simulink model "gm_fourxfour_designfxdpt_givens_vnl"  (R2018b)
settings: Solver=FixedStepDiscrete  StartTime=0.0  StopTime=0.18e-6  RelTol=1e-3
InitFcn:
  | if isempty(which('mylib'))
  |      tmp = fileparts(which(bdroot));
  |      run(fullfile(fileparts(tmp), '5-Utilities', 'addPathsPfcHw.m'));
  | end
  | 
  | data_types_givens
StopFcn:
  | GivensSim_Stop
undefined symbols (not defined in the file or in its folder): f
libraries: simulink x28, mylib x14
(part 2 of 4)

== system gm_fourxfour_designfxdpt_givens_vnl/Compare/Assert_R_11_i ==
  cosim : Inport
  dut : Inport  Port=2
  AssertEq : Assertion  StopWhenAssertionFail=off
  Compare To Zero : simulink/Logic and Bit Operations/Compare To Zero  relop===  OutDataTypeStr=boolean
  Relational Operator : RelationalOperator  Operator===  OutDataTypeStr=boolean  RndMeth=Nearest
  compare: R_11_i : Scope  NumInputPorts=3
  wires:
  Compare To Zero/1 -> compare: R_11_i/3  "err"
  Relational Operator/1 -> Compare To Zero/1, AssertEq/1
  cosim/1 -> compare: R_11_i/1, Relational Operator/1  "cosim"
  dut/1 -> compare: R_11_i/2, Relational Operator/2  "dut ref"

== system gm_fourxfour_designfxdpt_givens_vnl/Compare/Assert_R_11_r ==
  cosim : Inport
  dut : Inport  Port=2
  AssertEq : Assertion  StopWhenAssertionFail=off
  Compare To Zero : simulink/Logic and Bit Operations/Compare To Zero  relop===  OutDataTypeStr=boolean
  Relational Operator : RelationalOperator  Operator===  OutDataTypeStr=boolean  RndMeth=Nearest
  compare: R_11_r : Scope  NumInputPorts=3
  wires:
  Compare To Zero/1 -> compare: R_11_r/3  "err"
  Relational Operator/1 -> Compare To Zero/1, AssertEq/1
  cosim/1 -> compare: R_11_r/1, Relational Operator/1  "cosim"
  dut/1 -> compare: R_11_r/2, Relational Operator/2  "dut ref"

== system gm_fourxfour_designfxdpt_givens_vnl/Compare/Assert_R_12_i ==
  cosim : Inport
  dut : Inport  Port=2
  AssertEq : Assertion  StopWhenAssertionFail=off
  Compare To Zero : simulink/Logic and Bit Operations/Compare To Zero  relop===  OutDataTypeStr=boolean
  Relational Operator : RelationalOperator  Operator===  OutDataTypeStr=boolean  RndMeth=Nearest
  compare: R_12_i : Scope  NumInputPorts=3
  wires:
  Compare To Zero/1 -> compare: R_12_i/3  "err"
  Relational Operator/1 -> Compare To Zero/1, AssertEq/1
  cosim/1 -> compare: R_12_i/1, Relational Operator/1  "cosim"
  dut/1 -> compare: R_12_i/2, Relational Operator/2  "dut ref"

== system gm_fourxfour_designfxdpt_givens_vnl/Compare/Assert_R_12_r ==
  cosim : Inport
  dut : Inport  Port=2
  AssertEq : Assertion  StopWhenAssertionFail=off
  Compare To Zero : simulink/Logic and Bit Operations/Compare To Zero  relop===  OutDataTypeStr=boolean
  Relational Operator : RelationalOperator  Operator===  OutDataTypeStr=boolean  RndMeth=Nearest
  compare: R_12_r : Scope  NumInputPorts=3
  wires:
  Compare To Zero/1 -> compare: R_12_r/3  "err"
  Relational Operator/1 -> Compare To Zero/1, AssertEq/1
  cosim/1 -> compare: R_12_r/1, Relational Operator/1  "cosim"
  dut/1 -> compare: R_12_r/2, Relational Operator/2  "dut ref"

== system gm_fourxfour_designfxdpt_givens_vnl/Compare/Assert_R_13_i ==
  cosim : Inport
  dut : Inport  Port=2
  AssertEq : Assertion  StopWhenAssertionFail=off
  Compare To Zero : simulink/Logic and Bit Operations/Compare To Zero  relop===  OutDataTypeStr=boolean
  Relational Operator : RelationalOperator  Operator===  OutDataTypeStr=boolean  RndMeth=Nearest
  compare: R_13_i : Scope  NumInputPorts=3
  wires:
  Compare To Zero/1 -> compare: R_13_i/3  "err"
  Relational Operator/1 -> Compare To Zero/1, AssertEq/1
  cosim/1 -> compare: R_13_i/1, Relational Operator/1  "cosim"
  dut/1 -> compare: R_13_i/2, Relational Operator/2  "dut ref"

== system gm_fourxfour_designfxdpt_givens_vnl/Compare/Assert_R_13_r ==
  cosim : Inport
  dut : Inport  Port=2
  AssertEq : Assertion  StopWhenAssertionFail=off
  Compare To Zero : simulink/Logic and Bit Operations/Compare To Zero  relop===  OutDataTypeStr=boolean
  Relational Operator : RelationalOperator  Operator===  OutDataTypeStr=boolean  RndMeth=Nearest
  compare: R_13_r : Scope  NumInputPorts=3
  wires:
  Compare To Zero/1 -> compare: R_13_r/3  "err"
  Relational Operator/1 -> Compare To Zero/1, AssertEq/1
  cosim/1 -> compare: R_13_r/1, Relational Operator/1  "cosim"
  dut/1 -> compare: R_13_r/2, Relational Operator/2  "dut ref"

== system gm_fourxfour_designfxdpt_givens_vnl/Compare/Assert_R_14_i ==
  cosim : Inport
  dut : Inport  Port=2
  AssertEq : Assertion  StopWhenAssertionFail=off
  Compare To Zero : simulink/Logic and Bit Operations/Compare To Zero  relop===  OutDataTypeStr=boolean
  Relational Operator : RelationalOperator  Operator===  OutDataTypeStr=boolean  RndMeth=Nearest
  compare: R_14_i : Scope  NumInputPorts=3
  wires:
  Compare To Zero/1 -> compare: R_14_i/3  "err"
  Relational Operator/1 -> Compare To Zero/1, AssertEq/1
  cosim/1 -> compare: R_14_i/1, Relational Operator/1  "cosim"
  dut/1 -> compare: R_14_i/2, Relational Operator/2  "dut ref"

== system gm_fourxfour_designfxdpt_givens_vnl/Compare/Assert_R_14_r ==
  cosim : Inport
  dut : Inport  Port=2
  AssertEq : Assertion  StopWhenAssertionFail=off
  Compare To Zero : simulink/Logic and Bit Operations/Compare To Zero  relop===  OutDataTypeStr=boolean
  Relational Operator : RelationalOperator  Operator===  OutDataTypeStr=boolean  RndMeth=Nearest
  compare: R_14_r : Scope  NumInputPorts=3
  wires:
  Compare To Zero/1 -> compare: R_14_r/3  "err"
  Relational Operator/1 -> Compare To Zero/1, AssertEq/1
  cosim/1 -> compare: R_14_r/1, Relational Operator/1  "cosim"
  dut/1 -> compare: R_14_r/2, Relational Operator/2  "dut ref"

== system gm_fourxfour_designfxdpt_givens_vnl/Compare/Assert_R_22_i ==
  cosim : Inport
  dut : Inport  Port=2
  AssertEq : Assertion  StopWhenAssertionFail=off
  Compare To Zero : simulink/Logic and Bit Operations/Compare To Zero  relop===  OutDataTypeStr=boolean
  Relational Operator : RelationalOperator  Operator===  OutDataTypeStr=boolean  RndMeth=Nearest
  compare: R_22_i : Scope  NumInputPorts=3
  wires:
  Compare To Zero/1 -> compare: R_22_i/3  "err"
  Relational Operator/1 -> Compare To Zero/1, AssertEq/1
  cosim/1 -> compare: R_22_i/1, Relational Operator/1  "cosim"
  dut/1 -> compare: R_22_i/2, Relational Operator/2  "dut ref"

== system gm_fourxfour_designfxdpt_givens_vnl/Compare/Assert_R_22_r ==
  cosim : Inport
  dut : Inport  Port=2
  AssertEq : Assertion  StopWhenAssertionFail=off
  Compare To Zero : simulink/Logic and Bit Operations/Compare To Zero  relop===  OutDataTypeStr=boolean
  Relational Operator : RelationalOperator  Operator===  OutDataTypeStr=boolean  RndMeth=Nearest
  compare: R_22_r : Scope  NumInputPorts=3
  wires:
  Compare To Zero/1 -> compare: R_22_r/3  "err"
  Relational Operator/1 -> Compare To Zero/1, AssertEq/1
  cosim/1 -> compare: R_22_r/1, Relational Operator/1  "cosim"
  dut/1 -> compare: R_22_r/2, Relational Operator/2  "dut ref"

== system gm_fourxfour_designfxdpt_givens_vnl/Compare/Assert_R_23_i ==
  cosim : Inport
  dut : Inport  Port=2
  AssertEq : Assertion  StopWhenAssertionFail=off
  Compare To Zero : simulink/Logic and Bit Operations/Compare To Zero  relop===  OutDataTypeStr=boolean
  Relational Operator : RelationalOperator  Operator===  OutDataTypeStr=boolean  RndMeth=Nearest
  compare: R_23_i : Scope  NumInputPorts=3
  wires:
  Compare To Zero/1 -> compare: R_23_i/3  "err"
  Relational Operator/1 -> Compare To Zero/1, AssertEq/1
  cosim/1 -> compare: R_23_i/1, Relational Operator/1  "cosim"
  dut/1 -> compare: R_23_i/2, Relational Operator/2  "dut ref"

== system gm_fourxfour_designfxdpt_givens_vnl/Compare/Assert_R_23_r ==
  cosim : Inport
  dut : Inport  Port=2
  AssertEq : Assertion  StopWhenAssertionFail=off
  Compare To Zero : simulink/Logic and Bit Operations/Compare To Zero  relop===  OutDataTypeStr=boolean
  Relational Operator : RelationalOperator  Operator===  OutDataTypeStr=boolean  RndMeth=Nearest
  compare: R_23_r : Scope  NumInputPorts=3
  wires:
  Compare To Zero/1 -> compare: R_23_r/3  "err"
  Relational Operator/1 -> Compare To Zero/1, AssertEq/1
  cosim/1 -> compare: R_23_r/1, Relational Operator/1  "cosim"
  dut/1 -> compare: R_23_r/2, Relational Operator/2  "dut ref"

== system gm_fourxfour_designfxdpt_givens_vnl/Compare/Assert_R_24_i ==
  cosim : Inport
  dut : Inport  Port=2
  AssertEq : Assertion  StopWhenAssertionFail=off
  Compare To Zero : simulink/Logic and Bit Operations/Compare To Zero  relop===  OutDataTypeStr=boolean
  Relational Operator : RelationalOperator  Operator===  OutDataTypeStr=boolean  RndMeth=Nearest
  compare: R_24_i : Scope  NumInputPorts=3
  wires:
  Compare To Zero/1 -> compare: R_24_i/3  "err"
  Relational Operator/1 -> Compare To Zero/1, AssertEq/1
  cosim/1 -> compare: R_24_i/1, Relational Operator/1  "cosim"
  dut/1 -> compare: R_24_i/2, Relational Operator/2  "dut ref"

== system gm_fourxfour_designfxdpt_givens_vnl/Compare/Assert_R_24_r ==
  cosim : Inport
  dut : Inport  Port=2
  AssertEq : Assertion  StopWhenAssertionFail=off
  Compare To Zero : simulink/Logic and Bit Operations/Compare To Zero  relop===  OutDataTypeStr=boolean
  Relational Operator : RelationalOperator  Operator===  OutDataTypeStr=boolean  RndMeth=Nearest
  compare: R_24_r : Scope  NumInputPorts=3
  wires:
  Compare To Zero/1 -> compare: R_24_r/3  "err"
  Relational Operator/1 -> Compare To Zero/1, AssertEq/1
  cosim/1 -> compare: R_24_r/1, Relational Operator/1  "cosim"
  dut/1 -> compare: R_24_r/2, Relational Operator/2  "dut ref"

== system gm_fourxfour_designfxdpt_givens_vnl/Compare/Assert_R_33_i ==
  cosim : Inport
  dut : Inport  Port=2
  AssertEq : Assertion  StopWhenAssertionFail=off
  Compare To Zero : simulink/Logic and Bit Operations/Compare To Zero  relop===  OutDataTypeStr=boolean
  Relational Operator : RelationalOperator  Operator===  OutDataTypeStr=boolean  RndMeth=Nearest
  compare: R_33_i : Scope  NumInputPorts=3
  wires:
  Compare To Zero/1 -> compare: R_33_i/3  "err"
  Relational Operator/1 -> Compare To Zero/1, AssertEq/1
  cosim/1 -> compare: R_33_i/1, Relational Operator/1  "cosim"
  dut/1 -> compare: R_33_i/2, Relational Operator/2  "dut ref"

== system gm_fourxfour_designfxdpt_givens_vnl/Compare/Assert_R_33_r ==
  cosim : Inport
  dut : Inport  Port=2
  AssertEq : Assertion  StopWhenAssertionFail=off
  Compare To Zero : simulink/Logic and Bit Operations/Compare To Zero  relop===  OutDataTypeStr=boolean
  Relational Operator : RelationalOperator  Operator===  OutDataTypeStr=boolean  RndMeth=Nearest
  compare: R_33_r : Scope  NumInputPorts=3
  wires:
  Compare To Zero/1 -> compare: R_33_r/3  "err"
  Relational Operator/1 -> Compare To Zero/1, AssertEq/1
  cosim/1 -> compare: R_33_r/1, Relational Operator/1  "cosim"
  dut/1 -> compare: R_33_r/2, Relational Operator/2  "dut ref"

== system gm_fourxfour_designfxdpt_givens_vnl/Compare/Assert_R_34_i ==
  cosim : Inport
  dut : Inport  Port=2
  AssertEq : Assertion  StopWhenAssertionFail=off
  Compare To Zero : simulink/Logic and Bit Operations/Compare To Zero  relop===  OutDataTypeStr=boolean
  Relational Operator : RelationalOperator  Operator===  OutDataTypeStr=boolean  RndMeth=Nearest
  compare: R_34_i : Scope  NumInputPorts=3
  wires:
  Compare To Zero/1 -> compare: R_34_i/3  "err"
  Relational Operator/1 -> Compare To Zero/1, AssertEq/1
  cosim/1 -> compare: R_34_i/1, Relational Operator/1  "cosim"
  dut/1 -> compare: R_34_i/2, Relational Operator/2  "dut ref"

== system gm_fourxfour_designfxdpt_givens_vnl/Compare/Assert_R_34_r ==
  cosim : Inport
  dut : Inport  Port=2
  AssertEq : Assertion  StopWhenAssertionFail=off
  Compare To Zero : simulink/Logic and Bit Operations/Compare To Zero  relop===  OutDataTypeStr=boolean
  Relational Operator : RelationalOperator  Operator===  OutDataTypeStr=boolean  RndMeth=Nearest
  compare: R_34_r : Scope  NumInputPorts=3
  wires:
  Compare To Zero/1 -> compare: R_34_r/3  "err"
  Relational Operator/1 -> Compare To Zero/1, AssertEq/1
  cosim/1 -> compare: R_34_r/1, Relational Operator/1  "cosim"
  dut/1 -> compare: R_34_r/2, Relational Operator/2  "dut ref"

== system gm_fourxfour_designfxdpt_givens_vnl/Compare/Assert_R_44_i ==
  cosim : Inport
  dut : Inport  Port=2
  AssertEq : Assertion  StopWhenAssertionFail=off
  Compare To Zero : simulink/Logic and Bit Operations/Compare To Zero  relop===  OutDataTypeStr=boolean
  Relational Operator : RelationalOperator  Operator===  OutDataTypeStr=boolean  RndMeth=Nearest
  compare: R_44_i : Scope  NumInputPorts=3
  wires:
  Compare To Zero/1 -> compare: R_44_i/3  "err"
  Relational Operator/1 -> Compare To Zero/1, AssertEq/1
  cosim/1 -> compare: R_44_i/1, Relational Operator/1  "cosim"
  dut/1 -> compare: R_44_i/2, Relational Operator/2  "dut ref"

== system gm_fourxfour_designfxdpt_givens_vnl/Compare/Assert_R_44_r ==
  cosim : Inport
  dut : Inport  Port=2
  AssertEq : Assertion  StopWhenAssertionFail=off
  Compare To Zero : simulink/Logic and Bit Operations/Compare To Zero  relop===  OutDataTypeStr=boolean
  Relational Operator : RelationalOperator  Operator===  OutDataTypeStr=boolean  RndMeth=Nearest
  compare: R_44_r : Scope  NumInputPorts=3
  wires:
  Compare To Zero/1 -> compare: R_44_r/3  "err"
  Relational Operator/1 -> Compare To Zero/1, AssertEq/1
  cosim/1 -> compare: R_44_r/1, Relational Operator/1  "cosim"
  dut/1 -> compare: R_44_r/2, Relational Operator/2  "dut ref"

== system gm_fourxfour_designfxdpt_givens_vnl/Compare/Assert_bouti_1 ==
  cosim : Inport
  dut : Inport  Port=2
  AssertEq : Assertion  StopWhenAssertionFail=off
  Compare To Zero : simulink/Logic and Bit Operations/Compare To Zero  relop===  OutDataTypeStr=boolean
  Relational Operator : RelationalOperator  Operator===  OutDataTypeStr=boolean  RndMeth=Nearest
  compare: bouti_1 : Scope  NumInputPorts=3
  wires:
  Compare To Zero/1 -> compare: bouti_1/3  "err"
  Relational Operator/1 -> Compare To Zero/1, AssertEq/1
  cosim/1 -> compare: bouti_1/1, Relational Operator/1  "cosim"
  dut/1 -> compare: bouti_1/2, Relational Operator/2  "dut ref"

== system gm_fourxfour_designfxdpt_givens_vnl/Compare/Assert_bouti_2 ==
  cosim : Inport
  dut : Inport  Port=2
  AssertEq : Assertion  StopWhenAssertionFail=off
  Compare To Zero : simulink/Logic and Bit Operations/Compare To Zero  relop===  OutDataTypeStr=boolean
  Relational Operator : RelationalOperator  Operator===  OutDataTypeStr=boolean  RndMeth=Nearest
  compare: bouti_2 : Scope  NumInputPorts=3
  wires:
  Compare To Zero/1 -> compare: bouti_2/3  "err"
  Relational Operator/1 -> Compare To Zero/1, AssertEq/1
  cosim/1 -> compare: bouti_2/1, Relational Operator/1  "cosim"
  dut/1 -> compare: bouti_2/2, Relational Operator/2  "dut ref"

== system gm_fourxfour_designfxdpt_givens_vnl/Compare/Assert_bouti_3 ==
  cosim : Inport
  dut : Inport  Port=2
  AssertEq : Assertion  StopWhenAssertionFail=off
  Compare To Zero : simulink/Logic and Bit Operations/Compare To Zero  relop===  OutDataTypeStr=boolean
  Relational Operator : RelationalOperator  Operator===  OutDataTypeStr=boolean  RndMeth=Nearest
  compare: bouti_3 : Scope  NumInputPorts=3
  wires:
  Compare To Zero/1 -> compare: bouti_3/3  "err"
  Relational Operator/1 -> Compare To Zero/1, AssertEq/1
  cosim/1 -> compare: bouti_3/1, Relational Operator/1  "cosim"
  dut/1 -> compare: bouti_3/2, Relational Operator/2  "dut ref"

== system gm_fourxfour_designfxdpt_givens_vnl/Compare/Assert_bouti_4 ==
  cosim : Inport
  dut : Inport  Port=2
  AssertEq : Assertion  StopWhenAssertionFail=off
  Compare To Zero : simulink/Logic and Bit Operations/Compare To Zero  relop===  OutDataTypeStr=boolean
  Relational Operator : RelationalOperator  Operator===  OutDataTypeStr=boolean  RndMeth=Nearest
  compare: bouti_4 : Scope  NumInputPorts=3
  wires:
  Compare To Zero/1 -> compare: bouti_4/3  "err"
  Relational Operator/1 -> Compare To Zero/1, AssertEq/1
  cosim/1 -> compare: bouti_4/1, Relational Operator/1  "cosim"
  dut/1 -> compare: bouti_4/2, Relational Operator/2  "dut ref"

== system gm_fourxfour_designfxdpt_givens_vnl/Compare/Assert_boutr_1 ==
  cosim : Inport
  dut : Inport  Port=2
  AssertEq : Assertion  StopWhenAssertionFail=off
  Compare To Zero : simulink/Logic and Bit Operations/Compare To Zero  relop===  OutDataTypeStr=boolean
  Relational Operator : RelationalOperator  Operator===  OutDataTypeStr=boolean  RndMeth=Nearest
  compare: boutr_1 : Scope  NumInputPorts=3
  wires:
  Compare To Zero/1 -> compare: boutr_1/3  "err"
  Relational Operator/1 -> Compare To Zero/1, AssertEq/1
  cosim/1 -> compare: boutr_1/1, Relational Operator/1  "cosim"
  dut/1 -> compare: boutr_1/2, Relational Operator/2  "dut ref"

== system gm_fourxfour_designfxdpt_givens_vnl/Compare/Assert_boutr_2 ==
  cosim : Inport
  dut : Inport  Port=2
  AssertEq : Assertion  StopWhenAssertionFail=off
  Compare To Zero : simulink/Logic and Bit Operations/Compare To Zero  relop===  OutDataTypeStr=boolean
  Relational Operator : RelationalOperator  Operator===  OutDataTypeStr=boolean  RndMeth=Nearest
  compare: boutr_2 : Scope  NumInputPorts=3
  wires:
  Compare To Zero/1 -> compare: boutr_2/3  "err"
  Relational Operator/1 -> Compare To Zero/1, AssertEq/1
  cosim/1 -> compare: boutr_2/1, Relational Operator/1  "cosim"
  dut/1 -> compare: boutr_2/2, Relational Operator/2  "dut ref"

== system gm_fourxfour_designfxdpt_givens_vnl/Compare/Assert_boutr_3 ==
  cosim : Inport
  dut : Inport  Port=2
  AssertEq : Assertion  StopWhenAssertionFail=off
  Compare To Zero : simulink/Logic and Bit Operations/Compare To Zero  relop===  OutDataTypeStr=boolean
  Relational Operator : RelationalOperator  Operator===  OutDataTypeStr=boolean  RndMeth=Nearest
  compare: boutr_3 : Scope  NumInputPorts=3
  wires:
  Compare To Zero/1 -> compare: boutr_3/3  "err"
  Relational Operator/1 -> Compare To Zero/1, AssertEq/1
  cosim/1 -> compare: boutr_3/1, Relational Operator/1  "cosim"
  dut/1 -> compare: boutr_3/2, Relational Operator/2  "dut ref"

== system gm_fourxfour_designfxdpt_givens_vnl/Compare/Assert_boutr_4 ==
  cosim : Inport
  dut : Inport  Port=2
  AssertEq : Assertion  StopWhenAssertionFail=off
  Compare To Zero : simulink/Logic and Bit Operations/Compare To Zero  relop===  OutDataTypeStr=boolean
  Relational Operator : RelationalOperator  Operator===  OutDataTypeStr=boolean  RndMeth=Nearest
  compare: boutr_4 : Scope  NumInputPorts=3
  wires:
  Compare To Zero/1 -> compare: boutr_4/3  "err"
  Relational Operator/1 -> Compare To Zero/1, AssertEq/1
  cosim/1 -> compare: boutr_4/1, Relational Operator/1  "cosim"
  dut/1 -> compare: boutr_4/2, Relational Operator/2  "dut ref"

== system gm_fourxfour_designfxdpt_givens_vnl/Compare/CleanupScopes ==

== system gm_fourxfour_designfxdpt_givens_vnl/Compare/Enable ==

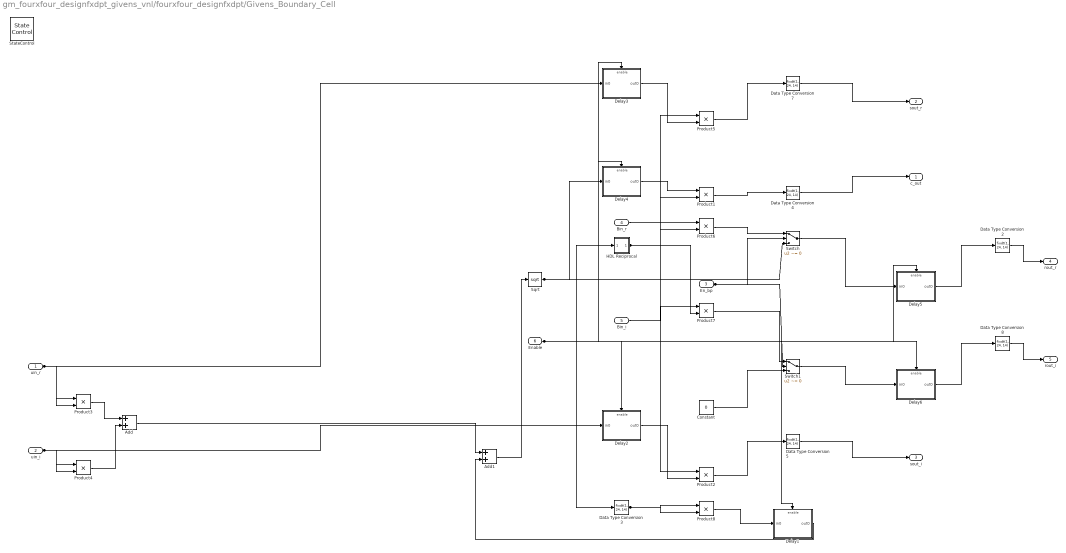
== system gm_fourxfour_designfxdpt_givens_vnl/fourxfour_designfxdpt/Givens_Boundary_Cell ==
  uin_r : Inport  OutDataTypeStr=fixdt(1, 24, 14)  SampleTime=1e-08
  uin_i : Inport  Port=2  OutDataTypeStr=fixdt(1, 24, 14)  SampleTime=1e-08
  En_bp : Inport  Port=3  OutDataTypeStr=boolean  SampleTime=1e-08
  Bin_r : Inport  Port=4  OutDataTypeStr=fixdt(1, 24, 14)  SampleTime=1e-08
  Bin_i : Inport  Port=5  OutDataTypeStr=fixdt(1, 24, 14)  SampleTime=1e-08
  Enable : Inport  Port=6  OutDataTypeStr=boolean  SampleTime=1e-08
  Add : Sum  AccumDataTypeStr=fixdt(1, 49, 28)  OutDataTypeStr=fixdt(1, 49, 28)  SampleTime=1e-08
  Add1 : Sum  AccumDataTypeStr=fixdt(1, 50, 28)  OutDataTypeStr=fixdt(0, 49, 28)  SampleTime=1e-08
  Constant : Constant  Value=0  OutDataTypeStr=fixdt(1, 24, 14)  SampleTime=-1
  Data Type Conversion{2..5,7..8} (6 alike) : DataTypeConversion  OutDataTypeStr=fixdt(1, 24, 14)  SampleTime=1e-08
  Delay1 : Subsystem
      settings: MinAlgLoopOccurrences=on
  Delay2 : Subsystem
      settings: MinAlgLoopOccurrences=on
  Delay3 : Subsystem
      settings: MinAlgLoopOccurrences=on
  Delay4 : Subsystem
      settings: MinAlgLoopOccurrences=on
  Delay5 : Subsystem
      settings: MinAlgLoopOccurrences=on
  Delay6 : Subsystem
      settings: MinAlgLoopOccurrences=on
  HDL Reciprocal : Subsystem
  Product1 : Product  Inputs=**  OutDataTypeStr=fixdt(0, 98, 48)  SampleTime=1e-08
  Product{2,5..7} (4 alike) : Product  Inputs=**  OutDataTypeStr=fixdt(1, 73, 34)  SampleTime=1e-08
  Product3 : Product  Inputs=**  OutDataTypeStr=fixdt(1, 48, 28)  SampleTime=1e-08
  Product4 : Product  Inputs=**  OutDataTypeStr=fixdt(1, 48, 28)  SampleTime=1e-08
  Product8 : Product  Inputs=**  OutDataTypeStr=fixdt(1, 48, 28)  SampleTime=1e-08
  Sqrt : Sqrt  OutputSignalType=real  SaturateOnIntegerOverflow=on
  StateControl : StateControl  StateControl=Synchronous
  Switch : Switch  Criteria=u2 ~= 0  Threshold=double(0)  OutDataTypeStr=fixdt(1, 73, 34)  SampleTime=1e-08
  Switch1 : Switch  Criteria=u2 ~= 0  Threshold=double(0)  OutDataTypeStr=fixdt(1, 73, 34)  SampleTime=1e-08
  c_out : Outport  InitialOutput=0
  sout_r : Outport  Port=2  InitialOutput=0
  sout_i : Outport  Port=3  InitialOutput=0
  rout_r : Outport  Port=4  InitialOutput=0
  rout_i : Outport  Port=5  InitialOutput=0
  wires:
  Switch1/1 -> Delay6/1(in0)
  Switch/1 -> Delay5/1(in0)
  Sqrt/1 -> Delay4/1(in0), Data Type Conversion3/1, HDL Reciprocal/1(In1), Switch/3
  Product8/1 -> Delay1/1(in0)
  Product7/1 -> Switch1/1
  Product6/1 -> Switch/1
  Product5/1 -> Data Type Conversion7/1
  Product4/1 -> Add/2
  Product3/1 -> Add/1
  Product2/1 -> Data Type Conversion5/1
  Product1/1 -> Data Type Conversion4/1
  HDL Reciprocal/1(Out1) -> Product1/2, Product2/1, Product5/1, Product6/2, Product7/2
  Delay6/1(out0) -> Data Type Conversion8/1
  Delay5/1(out0) -> Data Type Conversion2/1
  Delay4/1(out0) -> Product1/1
  Delay3/1(out0) -> Product5/2
  Delay2/1(out0) -> Product2/2
  Delay1/1(out0) -> Add1/2
  Data Type Conversion8/1 -> rout_i/1
  Data Type Conversion7/1 -> sout_r/1
  Data Type Conversion5/1 -> sout_i/1
  Data Type Conversion4/1 -> c_out/1
  Data Type Conversion3/1 -> Product8/1, Product8/2
  Data Type Conversion2/1 -> rout_r/1
  Constant/1 -> Switch1/3
  Add1/1 -> Sqrt/1
  Add/1 -> Add1/1
  Bin_i/1 -> Product7/1
  Bin_r/1 -> Product6/1
  En_bp/1 -> Switch/2, Switch1/2
  uin_i/1 -> Delay2/1(in0), Product4/1, Product4/2
  uin_r/1 -> Delay3/1(in0), Product3/1, Product3/2
  Enable/1 -> Delay1/Enable, Delay2/Enable, Delay3/Enable, Delay4/Enable, Delay5/Enable, Delay6/Enable

== system gm_fourxfour_designfxdpt_givens_vnl/fourxfour_designfxdpt/Givens_Boundary_Cell1 ==
  uin_r : Inport  OutDataTypeStr=fixdt(1, 24, 14)  SampleTime=1e-08
  uin_i : Inport  Port=2  OutDataTypeStr=fixdt(1, 24, 14)  SampleTime=1e-08
  En_bp : Inport  Port=3  OutDataTypeStr=boolean  SampleTime=1e-08
  Bin_r : Inport  Port=4  OutDataTypeStr=fixdt(1, 24, 14)  SampleTime=1e-08
  Bin_i : Inport  Port=5  OutDataTypeStr=fixdt(1, 24, 14)  SampleTime=1e-08
  Enable : Inport  Port=6  OutDataTypeStr=boolean  SampleTime=1e-08
  Add : Sum  AccumDataTypeStr=fixdt(1, 49, 28)  OutDataTypeStr=fixdt(1, 49, 28)  SampleTime=1e-08
  Add1 : Sum  AccumDataTypeStr=fixdt(1, 50, 28)  OutDataTypeStr=fixdt(0, 49, 28)  SampleTime=1e-08
  Constant : Constant  Value=0  OutDataTypeStr=fixdt(1, 24, 14)  SampleTime=-1
  Data Type Conversion{2..5,7..8} (6 alike) : DataTypeConversion  OutDataTypeStr=fixdt(1, 24, 14)  SampleTime=1e-08
  Delay1 : Subsystem
      settings: MinAlgLoopOccurrences=on
  Delay2 : Subsystem
      settings: MinAlgLoopOccurrences=on
  Delay3 : Subsystem
      settings: MinAlgLoopOccurrences=on
  Delay4 : Subsystem
      settings: MinAlgLoopOccurrences=on
  Delay5 : Subsystem
      settings: MinAlgLoopOccurrences=on
  Delay6 : Subsystem
      settings: MinAlgLoopOccurrences=on
  HDL Reciprocal : Subsystem
  Product1 : Product  Inputs=**  OutDataTypeStr=fixdt(0, 98, 48)  SampleTime=1e-08
  Product{2,5..7} (4 alike) : Product  Inputs=**  OutDataTypeStr=fixdt(1, 73, 34)  SampleTime=1e-08
  Product3 : Product  Inputs=**  OutDataTypeStr=fixdt(1, 48, 28)  SampleTime=1e-08
  Product4 : Product  Inputs=**  OutDataTypeStr=fixdt(1, 48, 28)  SampleTime=1e-08
  Product8 : Product  Inputs=**  OutDataTypeStr=fixdt(1, 48, 28)  SampleTime=1e-08
  Sqrt : Sqrt  OutputSignalType=real  SaturateOnIntegerOverflow=on
  StateControl : StateControl  StateControl=Synchronous
  Switch : Switch  Criteria=u2 ~= 0  Threshold=double(0)  OutDataTypeStr=fixdt(1, 73, 34)  SampleTime=1e-08
  Switch1 : Switch  Criteria=u2 ~= 0  Threshold=double(0)  OutDataTypeStr=fixdt(1, 73, 34)  SampleTime=1e-08
  c_out : Outport  InitialOutput=0
  sout_r : Outport  Port=2  InitialOutput=0
  sout_i : Outport  Port=3  InitialOutput=0
  rout_r : Outport  Port=4  InitialOutput=0
  rout_i : Outport  Port=5  InitialOutput=0
  wires:
  Switch1/1 -> Delay6/1(in0)
  Switch/1 -> Delay5/1(in0)
  Sqrt/1 -> Delay4/1(in0), Data Type Conversion3/1, HDL Reciprocal/1(In1), Switch/3
  Product8/1 -> Delay1/1(in0)
  Product7/1 -> Switch1/1
  Product6/1 -> Switch/1
  Product5/1 -> Data Type Conversion7/1
  Product4/1 -> Add/2
  Product3/1 -> Add/1
  Product2/1 -> Data Type Conversion5/1
  Product1/1 -> Data Type Conversion4/1
  HDL Reciprocal/1(Out1) -> Product1/2, Product2/1, Product5/1, Product6/2, Product7/2
  Delay6/1(out0) -> Data Type Conversion8/1
  Delay5/1(out0) -> Data Type Conversion2/1
  Delay4/1(out0) -> Product1/1
  Delay3/1(out0) -> Product5/2
  Delay2/1(out0) -> Product2/2
  Delay1/1(out0) -> Add1/2
  Data Type Conversion8/1 -> rout_i/1
  Data Type Conversion7/1 -> sout_r/1
  Data Type Conversion5/1 -> sout_i/1
  Data Type Conversion4/1 -> c_out/1
  Data Type Conversion3/1 -> Product8/1, Product8/2
  Data Type Conversion2/1 -> rout_r/1
  Constant/1 -> Switch1/3
  Add1/1 -> Sqrt/1
  Add/1 -> Add1/1
  Bin_i/1 -> Product7/1
  Bin_r/1 -> Product6/1
  En_bp/1 -> Switch/2, Switch1/2
  uin_i/1 -> Delay2/1(in0), Product4/1, Product4/2
  uin_r/1 -> Delay3/1(in0), Product3/1, Product3/2
  Enable/1 -> Delay1/Enable, Delay2/Enable, Delay3/Enable, Delay4/Enable, Delay5/Enable, Delay6/Enable

== system gm_fourxfour_designfxdpt_givens_vnl/fourxfour_designfxdpt/Givens_Boundary_Cell2 ==
  uin_r : Inport  OutDataTypeStr=fixdt(1, 24, 14)  SampleTime=1e-08
  uin_i : Inport  Port=2  OutDataTypeStr=fixdt(1, 24, 14)  SampleTime=1e-08
  En_bp : Inport  Port=3  OutDataTypeStr=boolean  SampleTime=1e-08
  Bin_r : Inport  Port=4  OutDataTypeStr=fixdt(1, 24, 14)  SampleTime=1e-08
  Bin_i : Inport  Port=5  OutDataTypeStr=fixdt(1, 24, 14)  SampleTime=1e-08
  Enable : Inport  Port=6  OutDataTypeStr=boolean  SampleTime=1e-08
  Add : Sum  AccumDataTypeStr=fixdt(1, 49, 28)  OutDataTypeStr=fixdt(1, 49, 28)  SampleTime=1e-08
  Add1 : Sum  AccumDataTypeStr=fixdt(1, 50, 28)  OutDataTypeStr=fixdt(0, 49, 28)  SampleTime=1e-08
  Constant : Constant  Value=0  OutDataTypeStr=fixdt(1, 24, 14)  SampleTime=-1
  Data Type Conversion{2..5,7..8} (6 alike) : DataTypeConversion  OutDataTypeStr=fixdt(1, 24, 14)  SampleTime=1e-08
  Delay1 : Subsystem
      settings: MinAlgLoopOccurrences=on
  Delay2 : Subsystem
      settings: MinAlgLoopOccurrences=on
  Delay3 : Subsystem
      settings: MinAlgLoopOccurrences=on
  Delay4 : Subsystem
      settings: MinAlgLoopOccurrences=on
  Delay5 : Subsystem
      settings: MinAlgLoopOccurrences=on
  Delay6 : Subsystem
      settings: MinAlgLoopOccurrences=on
  HDL Reciprocal : Subsystem
  Product1 : Product  Inputs=**  OutDataTypeStr=fixdt(0, 98, 48)  SampleTime=1e-08
  Product{2,5..7} (4 alike) : Product  Inputs=**  OutDataTypeStr=fixdt(1, 73, 34)  SampleTime=1e-08
  Product3 : Product  Inputs=**  OutDataTypeStr=fixdt(1, 48, 28)  SampleTime=1e-08
  Product4 : Product  Inputs=**  OutDataTypeStr=fixdt(1, 48, 28)  SampleTime=1e-08
  Product8 : Product  Inputs=**  OutDataTypeStr=fixdt(1, 48, 28)  SampleTime=1e-08
  Sqrt : Sqrt  OutputSignalType=real  SaturateOnIntegerOverflow=on
  StateControl : StateControl  StateControl=Synchronous
  Switch : Switch  Criteria=u2 ~= 0  Threshold=double(0)  OutDataTypeStr=fixdt(1, 73, 34)  SampleTime=1e-08
  Switch1 : Switch  Criteria=u2 ~= 0  Threshold=double(0)  OutDataTypeStr=fixdt(1, 73, 34)  SampleTime=1e-08
  c_out : Outport  InitialOutput=0
  sout_r : Outport  Port=2  InitialOutput=0
  sout_i : Outport  Port=3  InitialOutput=0
  rout_r : Outport  Port=4  InitialOutput=0
  rout_i : Outport  Port=5  InitialOutput=0
  wires:
  Switch1/1 -> Delay6/1(in0)
  Switch/1 -> Delay5/1(in0)
  Sqrt/1 -> Delay4/1(in0), Data Type Conversion3/1, HDL Reciprocal/1(In1), Switch/3
  Product8/1 -> Delay1/1(in0)
  Product7/1 -> Switch1/1
  Product6/1 -> Switch/1
  Product5/1 -> Data Type Conversion7/1
  Product4/1 -> Add/2
  Product3/1 -> Add/1
  Product2/1 -> Data Type Conversion5/1
  Product1/1 -> Data Type Conversion4/1
  HDL Reciprocal/1(Out1) -> Product1/2, Product2/1, Product5/1, Product6/2, Product7/2
  Delay6/1(out0) -> Data Type Conversion8/1
  Delay5/1(out0) -> Data Type Conversion2/1
  Delay4/1(out0) -> Product1/1
  Delay3/1(out0) -> Product5/2
  Delay2/1(out0) -> Product2/2
  Delay1/1(out0) -> Add1/2
  Data Type Conversion8/1 -> rout_i/1
  Data Type Conversion7/1 -> sout_r/1
  Data Type Conversion5/1 -> sout_i/1
  Data Type Conversion4/1 -> c_out/1
  Data Type Conversion3/1 -> Product8/1, Product8/2
  Data Type Conversion2/1 -> rout_r/1
  Constant/1 -> Switch1/3
  Add1/1 -> Sqrt/1
  Add/1 -> Add1/1
  Bin_i/1 -> Product7/1
  Bin_r/1 -> Product6/1
  En_bp/1 -> Switch/2, Switch1/2
  uin_i/1 -> Delay2/1(in0), Product4/1, Product4/2
  uin_r/1 -> Delay3/1(in0), Product3/1, Product3/2
  Enable/1 -> Delay1/Enable, Delay2/Enable, Delay3/Enable, Delay4/Enable, Delay5/Enable, Delay6/Enable

== system gm_fourxfour_designfxdpt_givens_vnl/fourxfour_designfxdpt/Givens_Boundary_Cell3 ==
  uin_r : Inport  OutDataTypeStr=fixdt(1, 24, 14)  SampleTime=1e-08
  uin_i : Inport  Port=2  OutDataTypeStr=fixdt(1, 24, 14)  SampleTime=1e-08
  En_bp : Inport  Port=3  OutDataTypeStr=boolean  SampleTime=1e-08
  Bin_r : Inport  Port=4  OutDataTypeStr=fixdt(1, 24, 14)  SampleTime=1e-08
  Bin_i : Inport  Port=5  OutDataTypeStr=fixdt(1, 24, 14)  SampleTime=1e-08
  Enable : Inport  Port=6  OutDataTypeStr=boolean  SampleTime=1e-08
  Add : Sum  AccumDataTypeStr=fixdt(1, 49, 28)  OutDataTypeStr=fixdt(1, 49, 28)  SampleTime=1e-08
  Add1 : Sum  AccumDataTypeStr=fixdt(1, 50, 28)  OutDataTypeStr=fixdt(0, 49, 28)  SampleTime=1e-08
  Constant : Constant  Value=0  OutDataTypeStr=fixdt(1, 24, 14)  SampleTime=-1
  Data Type Conversion{2..5,7..8} (6 alike) : DataTypeConversion  OutDataTypeStr=fixdt(1, 24, 14)  SampleTime=1e-08
  Delay1 : Subsystem
      settings: MinAlgLoopOccurrences=on
  Delay2 : Subsystem
      settings: MinAlgLoopOccurrences=on
  Delay3 : Subsystem
      settings: MinAlgLoopOccurrences=on
  Delay4 : Subsystem
      settings: MinAlgLoopOccurrences=on
  Delay5 : Subsystem
      settings: MinAlgLoopOccurrences=on
  Delay6 : Subsystem
      settings: MinAlgLoopOccurrences=on
  HDL Reciprocal : Subsystem
  Product1 : Product  Inputs=**  OutDataTypeStr=fixdt(0, 98, 48)  SampleTime=1e-08
  Product{2,5..7} (4 alike) : Product  Inputs=**  OutDataTypeStr=fixdt(1, 73, 34)  SampleTime=1e-08
  Product3 : Product  Inputs=**  OutDataTypeStr=fixdt(1, 48, 28)  SampleTime=1e-08
  Product4 : Product  Inputs=**  OutDataTypeStr=fixdt(1, 48, 28)  SampleTime=1e-08
  Product8 : Product  Inputs=**  OutDataTypeStr=fixdt(1, 48, 28)  SampleTime=1e-08
  Sqrt : Sqrt  OutputSignalType=real  SaturateOnIntegerOverflow=on
  StateControl : StateControl  StateControl=Synchronous
  Switch : Switch  Criteria=u2 ~= 0  Threshold=double(0)  OutDataTypeStr=fixdt(1, 73, 34)  SampleTime=1e-08
  Switch1 : Switch  Criteria=u2 ~= 0  Threshold=double(0)  OutDataTypeStr=fixdt(1, 73, 34)  SampleTime=1e-08
  c_out : Outport  InitialOutput=0
  sout_r : Outport  Port=2  InitialOutput=0
  sout_i : Outport  Port=3  InitialOutput=0
  rout_r : Outport  Port=4  InitialOutput=0
  rout_i : Outport  Port=5  InitialOutput=0
  wires:
  Switch1/1 -> Delay6/1(in0)
  Switch/1 -> Delay5/1(in0)
  Sqrt/1 -> Delay4/1(in0), Data Type Conversion3/1, HDL Reciprocal/1(In1), Switch/3
  Product8/1 -> Delay1/1(in0)
  Product7/1 -> Switch1/1
  Product6/1 -> Switch/1
  Product5/1 -> Data Type Conversion7/1
  Product4/1 -> Add/2
  Product3/1 -> Add/1
  Product2/1 -> Data Type Conversion5/1
  Product1/1 -> Data Type Conversion4/1
  HDL Reciprocal/1(Out1) -> Product1/2, Product2/1, Product5/1, Product6/2, Product7/2
  Delay6/1(out0) -> Data Type Conversion8/1
  Delay5/1(out0) -> Data Type Conversion2/1
  Delay4/1(out0) -> Product1/1
  Delay3/1(out0) -> Product5/2
  Delay2/1(out0) -> Product2/2
  Delay1/1(out0) -> Add1/2
  Data Type Conversion8/1 -> rout_i/1
  Data Type Conversion7/1 -> sout_r/1
  Data Type Conversion5/1 -> sout_i/1
  Data Type Conversion4/1 -> c_out/1
  Data Type Conversion3/1 -> Product8/1, Product8/2
  Data Type Conversion2/1 -> rout_r/1
  Constant/1 -> Switch1/3
  Add1/1 -> Sqrt/1
  Add/1 -> Add1/1
  Bin_i/1 -> Product7/1
  Bin_r/1 -> Product6/1
  En_bp/1 -> Switch/2, Switch1/2
  uin_i/1 -> Delay2/1(in0), Product4/1, Product4/2
  uin_r/1 -> Delay3/1(in0), Product3/1, Product3/2
  Enable/1 -> Delay1/Enable, Delay2/Enable, Delay3/Enable, Delay4/Enable, Delay5/Enable, Delay6/Enable

== system gm_fourxfour_designfxdpt_givens_vnl/fourxfour_designfxdpt/Givens_Internal_BW_Cell ==
  uin_r : Inport  OutDataTypeStr=fixdt(1, 24, 14)  SampleTime=1e-08
  uin_i : Inport  Port=2  OutDataTypeStr=fixdt(1, 24, 14)  SampleTime=1e-08
  cin : Inport  Port=3  OutDataTypeStr=fixdt(1, 24, 14)  SampleTime=1e-08
  sin_r : Inport  Port=4  OutDataTypeStr=fixdt(1, 24, 14)  SampleTime=1e-08
  sin_i : Inport  Port=5  OutDataTypeStr=fixdt(1, 24, 14)  SampleTime=1e-08
  Enable : Inport  Port=6  OutDataTypeStr=boolean  SampleTime=1e-08
  Add : Sum  Inputs=+-  AccumDataTypeStr=fixdt(1, 50, 28)  OutDataTypeStr=fixdt(1, 50, 28)  SampleTime=1e-08
  Add1 : Sum  Inputs=+-  AccumDataTypeStr=fixdt(1, 50, 28)  OutDataTypeStr=fixdt(1, 50, 28)  SampleTime=1e-08
  Data Type Conversion{8..11} (4 alike) : DataTypeConversion  OutDataTypeStr=fixdt(1, 24, 14)  SampleTime=1e-08
  Delay : Subsystem
      settings: MinAlgLoopOccurrences=on
  Delay1 : Subsystem
      settings: MinAlgLoopOccurrences=on
  StateControl : StateControl  StateControl=Synchronous
  Unary Minus : UnaryMinus  SampleTime=1e-08
  c*r_i : Product  Inputs=**  OutDataTypeStr=fixdt(1, 48, 28)  SampleTime=1e-08
  c*r_r : Product  Inputs=**  OutDataTypeStr=fixdt(1, 48, 28)  SampleTime=1e-08
  c*uin_i : Product  Inputs=**  OutDataTypeStr=fixdt(1, 48, 28)  SampleTime=1e-08
  c*uin_r : Product  Inputs=**  OutDataTypeStr=fixdt(1, 48, 28)  SampleTime=1e-08
  complex_mul : Subsystem
  complex_mul1 : Subsystem
  r_im : Sum  AccumDataTypeStr=fixdt(1, 50, 28)  OutDataTypeStr=fixdt(1, 50, 28)  SampleTime=1e-08
  r_r : Sum  AccumDataTypeStr=fixdt(1, 50, 28)  OutDataTypeStr=fixdt(1, 50, 28)  SampleTime=1e-08
  uout_r : Outport  InitialOutput=0
  uout_i : Outport  Port=2  InitialOutput=0
  cout : Outport  Port=3  InitialOutput=0
  sout_r : Outport  Port=4  InitialOutput=0
  sout_i : Outport  Port=5  InitialOutput=0
  rout_i : Outport  Port=6  InitialOutput=0
  rout_r : Outport  Port=7  InitialOutput=0
  wires:
  r_r/1 -> Data Type Conversion9/1
  r_im/1 -> Data Type Conversion8/1
  complex_mul1/2(Out1_i) -> r_im/1
  complex_mul1/1(Out1_r) -> r_r/1
  complex_mul/2(Out1_i) -> Add1/2
  complex_mul/1(Out1_r) -> Add/2
  c*uin_r/1 -> Add/1
  c*uin_i/1 -> Add1/1
  c*r_r/1 -> r_r/2
  c*r_i/1 -> r_im/2
  Unary Minus/1 -> complex_mul1/2(In1_i)
  Delay1/1(out0) -> complex_mul/3(In2_r), c*r_r/2
  Delay/1(out0) -> complex_mul/4(In2_i), c*r_i/2
  Data Type Conversion9/1 -> rout_r/1, Delay1/1(in0)
  Data Type Conversion8/1 -> rout_i/1, Delay/1(in0)
  Data Type Conversion11/1 -> uout_i/1
  Data Type Conversion10/1 -> uout_r/1
  Add1/1 -> Data Type Conversion11/1
  Add/1 -> Data Type Conversion10/1
  sin_i/1 -> sout_i/1, complex_mul/2(In1_i), Unary Minus/1
  sin_r/1 -> sout_r/1, complex_mul1/1(In1_r), complex_mul/1(In1_r)
  cin/1 -> cout/1, c*r_i/1, c*r_r/1, c*uin_i/1, c*uin_r/1
  uin_i/1 -> complex_mul1/4(In2_i), c*uin_i/2
  uin_r/1 -> complex_mul1/3(In2_r), c*uin_r/2
  Enable/1 -> Delay/Enable, Delay1/Enable

== system gm_fourxfour_designfxdpt_givens_vnl/fourxfour_designfxdpt/Givens_Internal_BW_Cell1 ==
  uin_r : Inport  OutDataTypeStr=fixdt(1, 24, 14)  SampleTime=1e-08
  uin_i : Inport  Port=2  OutDataTypeStr=fixdt(1, 24, 14)  SampleTime=1e-08
  cin : Inport  Port=3  OutDataTypeStr=fixdt(1, 24, 14)  SampleTime=1e-08
  sin_r : Inport  Port=4  OutDataTypeStr=fixdt(1, 24, 14)  SampleTime=1e-08
  sin_i : Inport  Port=5  OutDataTypeStr=fixdt(1, 24, 14)  SampleTime=1e-08
  Enable : Inport  Port=6  OutDataTypeStr=boolean  SampleTime=1e-08
  Add : Sum  Inputs=+-  AccumDataTypeStr=fixdt(1, 50, 28)  OutDataTypeStr=fixdt(1, 50, 28)  SampleTime=1e-08
  Add1 : Sum  Inputs=+-  AccumDataTypeStr=fixdt(1, 50, 28)  OutDataTypeStr=fixdt(1, 50, 28)  SampleTime=1e-08
  Data Type Conversion{8..11} (4 alike) : DataTypeConversion  OutDataTypeStr=fixdt(1, 24, 14)  SampleTime=1e-08
  Delay : Subsystem
      settings: MinAlgLoopOccurrences=on
  Delay1 : Subsystem
      settings: MinAlgLoopOccurrences=on
  StateControl : StateControl  StateControl=Synchronous
  Unary Minus : UnaryMinus  SampleTime=1e-08
  c*r_i : Product  Inputs=**  OutDataTypeStr=fixdt(1, 48, 28)  SampleTime=1e-08
  c*r_r : Product  Inputs=**  OutDataTypeStr=fixdt(1, 48, 28)  SampleTime=1e-08
  c*uin_i : Product  Inputs=**  OutDataTypeStr=fixdt(1, 48, 28)  SampleTime=1e-08
  c*uin_r : Product  Inputs=**  OutDataTypeStr=fixdt(1, 48, 28)  SampleTime=1e-08
  complex_mul : Subsystem
  complex_mul1 : Subsystem
  r_im : Sum  AccumDataTypeStr=fixdt(1, 50, 28)  OutDataTypeStr=fixdt(1, 50, 28)  SampleTime=1e-08
  r_r : Sum  AccumDataTypeStr=fixdt(1, 50, 28)  OutDataTypeStr=fixdt(1, 50, 28)  SampleTime=1e-08
  uout_r : Outport  InitialOutput=0
  uout_i : Outport  Port=2  InitialOutput=0
  cout : Outport  Port=3  InitialOutput=0
  sout_r : Outport  Port=4  InitialOutput=0
  sout_i : Outport  Port=5  InitialOutput=0
  rout_i : Outport  Port=6  InitialOutput=0
  rout_r : Outport  Port=7  InitialOutput=0
  wires:
  r_r/1 -> Data Type Conversion9/1
  r_im/1 -> Data Type Conversion8/1
  complex_mul1/2(Out1_i) -> r_im/1
  complex_mul1/1(Out1_r) -> r_r/1
  complex_mul/2(Out1_i) -> Add1/2
  complex_mul/1(Out1_r) -> Add/2
  c*uin_r/1 -> Add/1
  c*uin_i/1 -> Add1/1
  c*r_r/1 -> r_r/2
  c*r_i/1 -> r_im/2
  Unary Minus/1 -> complex_mul1/2(In1_i)
  Delay1/1(out0) -> complex_mul/3(In2_r), c*r_r/2
  Delay/1(out0) -> complex_mul/4(In2_i), c*r_i/2
  Data Type Conversion9/1 -> rout_r/1, Delay1/1(in0)
  Data Type Conversion8/1 -> rout_i/1, Delay/1(in0)
  Data Type Conversion11/1 -> uout_i/1
  Data Type Conversion10/1 -> uout_r/1
  Add1/1 -> Data Type Conversion11/1
  Add/1 -> Data Type Conversion10/1
  sin_i/1 -> sout_i/1, complex_mul/2(In1_i), Unary Minus/1
  sin_r/1 -> sout_r/1, complex_mul1/1(In1_r), complex_mul/1(In1_r)
  cin/1 -> cout/1, c*r_i/1, c*r_r/1, c*uin_i/1, c*uin_r/1
  uin_i/1 -> complex_mul1/4(In2_i), c*uin_i/2
  uin_r/1 -> complex_mul1/3(In2_r), c*uin_r/2
  Enable/1 -> Delay/Enable, Delay1/Enable

== system gm_fourxfour_designfxdpt_givens_vnl/fourxfour_designfxdpt/Givens_Internal_BW_Cell2 ==
  uin_r : Inport  OutDataTypeStr=fixdt(1, 24, 14)  SampleTime=1e-08
  uin_i : Inport  Port=2  OutDataTypeStr=fixdt(1, 24, 14)  SampleTime=1e-08
  cin : Inport  Port=3  OutDataTypeStr=fixdt(1, 24, 14)  SampleTime=1e-08
  sin_r : Inport  Port=4  OutDataTypeStr=fixdt(1, 24, 14)  SampleTime=1e-08
  sin_i : Inport  Port=5  OutDataTypeStr=fixdt(1, 24, 14)  SampleTime=1e-08
  Enable : Inport  Port=6  OutDataTypeStr=boolean  SampleTime=1e-08
  Add : Sum  Inputs=+-  AccumDataTypeStr=fixdt(1, 50, 28)  OutDataTypeStr=fixdt(1, 50, 28)  SampleTime=1e-08
  Add1 : Sum  Inputs=+-  AccumDataTypeStr=fixdt(1, 50, 28)  OutDataTypeStr=fixdt(1, 50, 28)  SampleTime=1e-08
  Data Type Conversion{8..11} (4 alike) : DataTypeConversion  OutDataTypeStr=fixdt(1, 24, 14)  SampleTime=1e-08
  Delay : Subsystem
      settings: MinAlgLoopOccurrences=on
  Delay1 : Subsystem
      settings: MinAlgLoopOccurrences=on
  StateControl : StateControl  StateControl=Synchronous
  Unary Minus : UnaryMinus  SampleTime=1e-08
  c*r_i : Product  Inputs=**  OutDataTypeStr=fixdt(1, 48, 28)  SampleTime=1e-08
  c*r_r : Product  Inputs=**  OutDataTypeStr=fixdt(1, 48, 28)  SampleTime=1e-08
  c*uin_i : Product  Inputs=**  OutDataTypeStr=fixdt(1, 48, 28)  SampleTime=1e-08
  c*uin_r : Product  Inputs=**  OutDataTypeStr=fixdt(1, 48, 28)  SampleTime=1e-08
  complex_mul : Subsystem
  complex_mul1 : Subsystem
  r_im : Sum  AccumDataTypeStr=fixdt(1, 50, 28)  OutDataTypeStr=fixdt(1, 50, 28)  SampleTime=1e-08
  r_r : Sum  AccumDataTypeStr=fixdt(1, 50, 28)  OutDataTypeStr=fixdt(1, 50, 28)  SampleTime=1e-08
  uout_r : Outport  InitialOutput=0
  uout_i : Outport  Port=2  InitialOutput=0
  cout : Outport  Port=3  InitialOutput=0
  sout_r : Outport  Port=4  InitialOutput=0
  sout_i : Outport  Port=5  InitialOutput=0
  rout_i : Outport  Port=6  InitialOutput=0
  rout_r : Outport  Port=7  InitialOutput=0
  wires:
  r_r/1 -> Data Type Conversion9/1
  r_im/1 -> Data Type Conversion8/1
  complex_mul1/2(Out1_i) -> r_im/1
  complex_mul1/1(Out1_r) -> r_r/1
  complex_mul/2(Out1_i) -> Add1/2
  complex_mul/1(Out1_r) -> Add/2
  c*uin_r/1 -> Add/1
  c*uin_i/1 -> Add1/1
  c*r_r/1 -> r_r/2
  c*r_i/1 -> r_im/2
  Unary Minus/1 -> complex_mul1/2(In1_i)
  Delay1/1(out0) -> complex_mul/3(In2_r), c*r_r/2
  Delay/1(out0) -> complex_mul/4(In2_i), c*r_i/2
  Data Type Conversion9/1 -> rout_r/1, Delay1/1(in0)
  Data Type Conversion8/1 -> rout_i/1, Delay/1(in0)
  Data Type Conversion11/1 -> uout_i/1
  Data Type Conversion10/1 -> uout_r/1
  Add1/1 -> Data Type Conversion11/1
  Add/1 -> Data Type Conversion10/1
  sin_i/1 -> sout_i/1, complex_mul/2(In1_i), Unary Minus/1
  sin_r/1 -> sout_r/1, complex_mul1/1(In1_r), complex_mul/1(In1_r)
  cin/1 -> cout/1, c*r_i/1, c*r_r/1, c*uin_i/1, c*uin_r/1
  uin_i/1 -> complex_mul1/4(In2_i), c*uin_i/2
  uin_r/1 -> complex_mul1/3(In2_r), c*uin_r/2
  Enable/1 -> Delay/Enable, Delay1/Enable

== system gm_fourxfour_designfxdpt_givens_vnl/fourxfour_designfxdpt/Givens_Internal_BW_Cell3 ==
  uin_r : Inport  OutDataTypeStr=fixdt(1, 24, 14)  SampleTime=1e-08
  uin_i : Inport  Port=2  OutDataTypeStr=fixdt(1, 24, 14)  SampleTime=1e-08
  cin : Inport  Port=3  OutDataTypeStr=fixdt(1, 24, 14)  SampleTime=1e-08
  sin_r : Inport  Port=4  OutDataTypeStr=fixdt(1, 24, 14)  SampleTime=1e-08
  sin_i : Inport  Port=5  OutDataTypeStr=fixdt(1, 24, 14)  SampleTime=1e-08
  Enable : Inport  Port=6  OutDataTypeStr=boolean  SampleTime=1e-08
  Add : Sum  Inputs=+-  AccumDataTypeStr=fixdt(1, 50, 28)  OutDataTypeStr=fixdt(1, 50, 28)  SampleTime=1e-08
  Add1 : Sum  Inputs=+-  AccumDataTypeStr=fixdt(1, 50, 28)  OutDataTypeStr=fixdt(1, 50, 28)  SampleTime=1e-08
  Data Type Conversion{8..11} (4 alike) : DataTypeConversion  OutDataTypeStr=fixdt(1, 24, 14)  SampleTime=1e-08
  Delay : Subsystem
      settings: MinAlgLoopOccurrences=on
  Delay1 : Subsystem
      settings: MinAlgLoopOccurrences=on
  StateControl : StateControl  StateControl=Synchronous
  Unary Minus : UnaryMinus  SampleTime=1e-08
  c*r_i : Product  Inputs=**  OutDataTypeStr=fixdt(1, 48, 28)  SampleTime=1e-08
  c*r_r : Product  Inputs=**  OutDataTypeStr=fixdt(1, 48, 28)  SampleTime=1e-08
  c*uin_i : Product  Inputs=**  OutDataTypeStr=fixdt(1, 48, 28)  SampleTime=1e-08
  c*uin_r : Product  Inputs=**  OutDataTypeStr=fixdt(1, 48, 28)  SampleTime=1e-08
  complex_mul : Subsystem
  complex_mul1 : Subsystem
  r_im : Sum  AccumDataTypeStr=fixdt(1, 50, 28)  OutDataTypeStr=fixdt(1, 50, 28)  SampleTime=1e-08
  r_r : Sum  AccumDataTypeStr=fixdt(1, 50, 28)  OutDataTypeStr=fixdt(1, 50, 28)  SampleTime=1e-08
  uout_r : Outport  InitialOutput=0
  uout_i : Outport  Port=2  InitialOutput=0
  cout : Outport  Port=3  InitialOutput=0
  sout_r : Outport  Port=4  InitialOutput=0
  sout_i : Outport  Port=5  InitialOutput=0
  rout_i : Outport  Port=6  InitialOutput=0
  rout_r : Outport  Port=7  InitialOutput=0
  wires:
  r_r/1 -> Data Type Conversion9/1
  r_im/1 -> Data Type Conversion8/1
  complex_mul1/2(Out1_i) -> r_im/1
  complex_mul1/1(Out1_r) -> r_r/1
  complex_mul/2(Out1_i) -> Add1/2
  complex_mul/1(Out1_r) -> Add/2
  c*uin_r/1 -> Add/1
  c*uin_i/1 -> Add1/1
  c*r_r/1 -> r_r/2
  c*r_i/1 -> r_im/2
  Unary Minus/1 -> complex_mul1/2(In1_i)
  Delay1/1(out0) -> complex_mul/3(In2_r), c*r_r/2
  Delay/1(out0) -> complex_mul/4(In2_i), c*r_i/2
  Data Type Conversion9/1 -> rout_r/1, Delay1/1(in0)
  Data Type Conversion8/1 -> rout_i/1, Delay/1(in0)
  Data Type Conversion11/1 -> uout_i/1
  Data Type Conversion10/1 -> uout_r/1
  Add1/1 -> Data Type Conversion11/1
  Add/1 -> Data Type Conversion10/1
  sin_i/1 -> sout_i/1, complex_mul/2(In1_i), Unary Minus/1
  sin_r/1 -> sout_r/1, complex_mul1/1(In1_r), complex_mul/1(In1_r)
  cin/1 -> cout/1, c*r_i/1, c*r_r/1, c*uin_i/1, c*uin_r/1
  uin_i/1 -> complex_mul1/4(In2_i), c*uin_i/2
  uin_r/1 -> complex_mul1/3(In2_r), c*uin_r/2
  Enable/1 -> Delay/Enable, Delay1/Enable

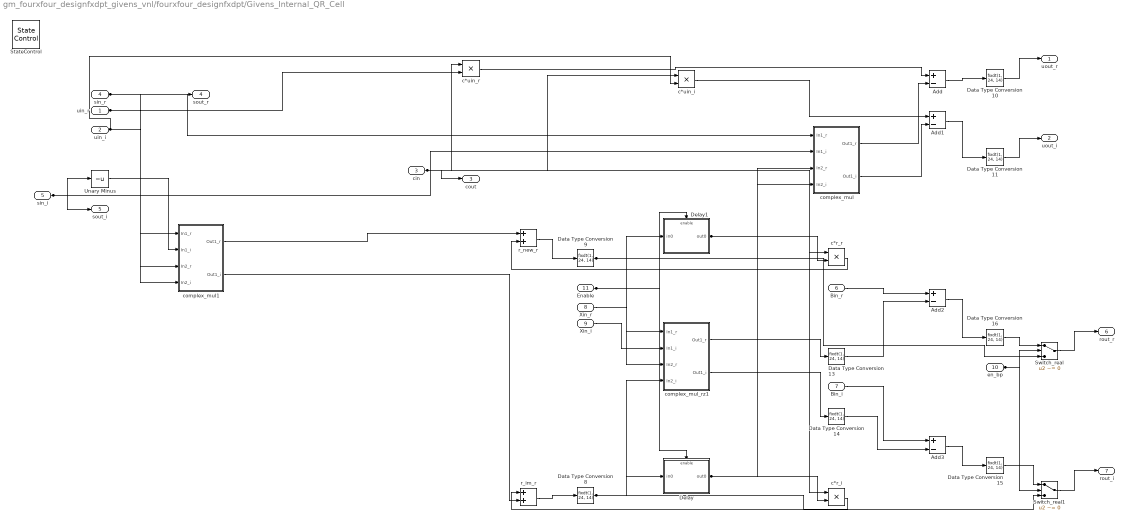
== system gm_fourxfour_designfxdpt_givens_vnl/fourxfour_designfxdpt/Givens_Internal_QR_Cell ==
  uin_r : Inport  OutDataTypeStr=fixdt(1, 24, 14)  SampleTime=1e-08
  uin_i : Inport  Port=2  OutDataTypeStr=fixdt(1, 24, 14)  SampleTime=1e-08
  cin : Inport  Port=3  OutDataTypeStr=fixdt(1, 24, 14)  SampleTime=1e-08
  sin_r : Inport  Port=4  OutDataTypeStr=fixdt(1, 24, 14)  SampleTime=1e-08
  sin_i : Inport  Port=5  OutDataTypeStr=fixdt(1, 24, 14)  SampleTime=1e-08
  Bin_r : Inport  Port=6  OutDataTypeStr=fixdt(1, 24, 14)  SampleTime=1e-08
  Bin_i : Inport  Port=7  OutDataTypeStr=fixdt(1, 24, 14)  SampleTime=1e-08
  Xin_r : Inport  Port=8  OutDataTypeStr=fixdt(1, 24, 14)  SampleTime=1e-08
  Xin_i : Inport  Port=9  OutDataTypeStr=fixdt(1, 24, 14)  SampleTime=1e-08
  en_bp : Inport  Port=10  OutDataTypeStr=boolean  SampleTime=1e-08
  Enable : Inport  Port=11  OutDataTypeStr=boolean  SampleTime=1e-08
  Add : Sum  Inputs=+-  AccumDataTypeStr=fixdt(1, 50, 28)  OutDataTypeStr=fixdt(1, 50, 28)  SampleTime=1e-08
  Add1 : Sum  Inputs=+-  AccumDataTypeStr=fixdt(1, 50, 28)  OutDataTypeStr=fixdt(1, 50, 28)  SampleTime=1e-08
  Add2 : Sum  Inputs=+-  AccumDataTypeStr=fixdt(1, 25, 14)  OutDataTypeStr=fixdt(1, 25, 14)  SampleTime=1e-08
  Add3 : Sum  Inputs=+-  AccumDataTypeStr=fixdt(1, 25, 14)  OutDataTypeStr=fixdt(1, 25, 14)  SampleTime=1e-08
  Data Type Conversion{8..11,13..16} (8 alike) : DataTypeConversion  OutDataTypeStr=fixdt(1, 24, 14)  SampleTime=1e-08
  Delay : Subsystem
      settings: MinAlgLoopOccurrences=on
  Delay1 : Subsystem
      settings: MinAlgLoopOccurrences=on
  StateControl : StateControl  StateControl=Synchronous
  Switch_real : Switch  Criteria=u2 ~= 0  Threshold=double(0)  OutDataTypeStr=fixdt(1, 24, 14)  SampleTime=1e-08
  Switch_real1 : Switch  Criteria=u2 ~= 0  Threshold=double(0)  OutDataTypeStr=fixdt(1, 24, 14)  SampleTime=1e-08
  Unary Minus : UnaryMinus  SampleTime=1e-08
  c*r_i : Product  Inputs=**  OutDataTypeStr=fixdt(1, 48, 28)  SampleTime=1e-08
  c*r_r : Product  Inputs=**  OutDataTypeStr=fixdt(1, 48, 28)  SampleTime=1e-08
  c*uin_i : Product  Inputs=**  OutDataTypeStr=fixdt(1, 48, 28)  SampleTime=1e-08
  c*uin_r : Product  Inputs=**  OutDataTypeStr=fixdt(1, 48, 28)  SampleTime=1e-08
  complex_mul : Subsystem
  complex_mul1 : Subsystem
  complex_mul_rz1 : Subsystem
  r_im_r : Sum  AccumDataTypeStr=fixdt(1, 50, 28)  OutDataTypeStr=fixdt(1, 50, 28)  SampleTime=1e-08
  r_new_r : Sum  AccumDataTypeStr=fixdt(1, 50, 28)  OutDataTypeStr=fixdt(1, 50, 28)  SampleTime=1e-08
  uout_r : Outport  InitialOutput=0
  uout_i : Outport  Port=2  InitialOutput=0
  cout : Outport  Port=3  InitialOutput=0
  sout_r : Outport  Port=4  InitialOutput=0
  sout_i : Outport  Port=5  InitialOutput=0
  rout_r : Outport  Port=6  InitialOutput=0
  rout_i : Outport  Port=7  InitialOutput=0
  wires:
  r_new_r/1 -> Data Type Conversion9/1
  r_im_r/1 -> Data Type Conversion8/1
  complex_mul_rz1/2(Out1_i) -> Data Type Conversion14/1
  complex_mul_rz1/1(Out1_r) -> Data Type Conversion13/1
  complex_mul1/2(Out1_i) -> r_im_r/2
  complex_mul1/1(Out1_r) -> r_new_r/1
  complex_mul/2(Out1_i) -> Add1/2
  complex_mul/1(Out1_r) -> Add/2
  c*uin_r/1 -> Add/1
  c*uin_i/1 -> Add1/1
  c*r_r/1 -> r_new_r/2
  c*r_i/1 -> r_im_r/1
  Unary Minus/1 -> complex_mul1/2(In1_i)
  Switch_real1/1 -> rout_i/1
  Switch_real/1 -> rout_r/1
  Delay1/1(out0) -> complex_mul/3(In2_r), c*r_r/2
  Delay/1(out0) -> complex_mul/4(In2_i), c*r_i/2
  Data Type Conversion9/1 -> complex_mul_rz1/3(In2_r), Delay1/1(in0), Switch_real/3
  Data Type Conversion8/1 -> complex_mul_rz1/4(In2_i), Delay/1(in0), Switch_real1/3
  Data Type Conversion16/1 -> Switch_real/1
  Data Type Conversion15/1 -> Switch_real1/1
  Data Type Conversion14/1 -> Add3/2
  Data Type Conversion13/1 -> Add2/2
  Data Type Conversion11/1 -> uout_i/1
  Data Type Conversion10/1 -> uout_r/1
  Add3/1 -> Data Type Conversion15/1
  Add2/1 -> Data Type Conversion16/1
  Add1/1 -> Data Type Conversion11/1
  Add/1 -> Data Type Conversion10/1
  en_bp/1 -> Switch_real/2, Switch_real1/2
  Xin_i/1 -> complex_mul_rz1/2(In1_i)
  Xin_r/1 -> complex_mul_rz1/1(In1_r)
  Bin_i/1 -> Add3/1
  Bin_r/1 -> Add2/1
  sin_i/1 -> sout_i/1, complex_mul/2(In1_i), Unary Minus/1
  sin_r/1 -> sout_r/1, complex_mul1/1(In1_r), complex_mul/1(In1_r)
  cin/1 -> cout/1, c*r_i/1, c*r_r/1, c*uin_i/1, c*uin_r/1
  uin_i/1 -> complex_mul1/4(In2_i), c*uin_i/2
  uin_r/1 -> complex_mul1/3(In2_r), c*uin_r/2
  Enable/1 -> Delay/Enable, Delay1/Enable
